simulink model "VMC_14Dof_2024a"  (R2024a)
settings: Solver=FixedStepDiscrete  StartTime=0.0  StopTime=10.0  FixedStep=0.001  RelTol=1e-3
InitFcn:
  | unlinear_14DOF_Parameters
undefined symbols (not defined in the file): Bf, Br, Cp_fl, Cp_fr, Cp_rl, Cp_rr, Cs_f, eta_FMotor, eta_RMotor, f, g, He, Hp, i_fa, i_ra, i_sw, I_tire, Ix, Iy, Iz, ks_f, kw, Lf, Lr, m, mb, mu, mw, r, Sampletime, Standstill_buffer, vx0, vxlim, w0
libraries: simulink x32, slpidlib x6
(part 2 of 5)

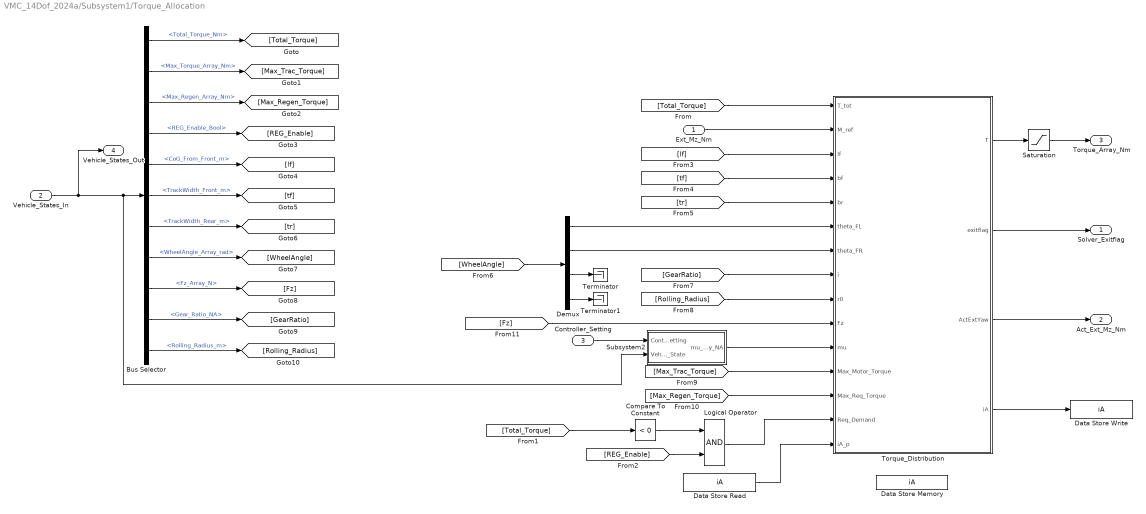
== system VMC_14Dof_2024a/Subsystem1/Torque_Allocation ==
  Ext_Mz_Nm : Inport
  Vehicle_States_In : Inport  Port=2
  Controller_Setting : Inport  Port=3
  Bus Selector : BusSelector  OutputSignals=Torque_Demand.Total_Torque_Nm,Torque_Demand.Max_Torque_Array_Nm,Torque_Demand.Max_Regen_Array_Nm,Torque_Demand.REG_Enable_Bool,Vehicle_Static_Parameter.CoG_From_Front_m,Vehicle_Static_Parameter.TrackWidth_Front_m,Vehicle_Static_Parameter.TrackWidth_Rear_m,WheelAngle.WheelAngle_Array_rad,Tire_Force.Fz_Array_N,Vehicle_Static_Parameter.Gear_Ratio_NA,Vehicle_Static_Parameter.Rolling_Radius_m
  Compare To Constant : simulink/Logic and Bit Operations/Compare To Constant  relop=<  const=0  OutDataTypeStr=boolean
  Data Store Memory : DataStoreMemory  DataStoreName=iA  WriteAfterWriteMsg=warning  InitialValue=[0,0,0,0,0,0,0,0]  ShowAdditionalParam=off  OutDataTypeStr=boolean
  Data Store Read : DataStoreRead  DataStoreName=iA  IndexOptions=Index vector (dialog)  Indices=1  OutputSizes=1
  Data Store Write : DataStoreWrite  DataStoreName=iA  IndexOptions=Index vector (dialog)  Indices=1  OutputSizes=1
  Demux : Demux
  Logical Operator : Logic  AllPortsSameDT=off  OutDataTypeStr=boolean
  Saturation : Saturate  UpperLimit=21  LowerLimit=-21
  Subsystem2 : Subsystem
  Terminator : Terminator
  Terminator1 : Terminator
  Torque_Distribution : MATLAB Function  TreatAsAtomicUnit=on
  Solver_Exitflag : Outport
  Act_Ext_Mz_Nm : Outport  Port=2
  Torque_Array_Nm : Outport  Port=3
  Vehicle_States_Out : Outport  Port=4
  wires:
  [Rolling_Radius] -> Torque_Distribution/9(r0)
  [tr] -> Torque_Distribution/5(br)
  [GearRatio] -> Torque_Distribution/8(i)
  [tf] -> Torque_Distribution/4(bf)
  [lf] -> Torque_Distribution/3(lf)
  [Max_Regen_Torque] -> Torque_Distribution/13(Max_Req_Torque)
  Torque_Distribution/2(exitflag) -> Solver_Exitflag/1
  Demux/1 -> Torque_Distribution/6(theta_FL)
  Demux/2 -> Torque_Distribution/7(theta_FR)
  [Fz] -> Torque_Distribution/10(Fz)
  [Max_Trac_Torque] -> Torque_Distribution/12(Max_Motor_Torque)
  Torque_Distribution/4(iA) -> Data Store Write/1
  Torque_Distribution/1(T) -> Saturation/1
  Data Store Read/1 -> Torque_Distribution/15(iA_p)
  Ext_Mz_Nm/1 -> Torque_Distribution/2(M_ref)
  Subsystem2/1(mu_x_Array_NA) -> Torque_Distribution/11(mu)
  Torque_Distribution/3(ActExtYaw) -> Act_Ext_Mz_Nm/1
  Logical Operator/1 -> Torque_Distribution/14(Req_Demand)
  Compare To Constant/1 -> Logical Operator/1
  [REG_Enable] -> Logical Operator/2
  Vehicle_States_In/1 -> Vehicle_States_Out/1, Subsystem2/2(Vehicle_State), Bus Selector/1
  Bus Selector/1 -> [Total_Torque]  "<Total_Torque_Nm>"
  Bus Selector/2 -> [Max_Trac_Torque]  "<Max_Torque_Array_Nm>"
  Bus Selector/3 -> [Max_Regen_Torque]  "<Max_Regen_Array_Nm>"
  Bus Selector/4 -> [REG_Enable]  "<REG_Enable_Bool>"
  Bus Selector/5 -> [lf]  "<CoG_From_Front_m>"
  Bus Selector/6 -> [tf]  "<TrackWidth_Front_m>"
  Bus Selector/7 -> [tr]  "<TrackWidth_Rear_m>"
  Bus Selector/8 -> [WheelAngle]  "<WheelAngle_Array_rad>"
  Bus Selector/9 -> [Fz]  "<Fz_Array_N>"
  Bus Selector/10 -> [GearRatio]  "<Gear_Ratio_NA>"
  Bus Selector/11 -> [Rolling_Radius]  "<Rolling_Radius_m>"
  [Total_Torque] -> Torque_Distribution/1(T_tot)
  [Total_Torque] -> Compare To Constant/1
  [WheelAngle] -> Demux/1
  Demux/3 -> Terminator/1
  Demux/4 -> Terminator1/1
  Controller_Setting/1 -> Subsystem2/1(Controller_Setting)
  Saturation/1 -> Torque_Array_Nm/1

== system VMC_14Dof_2024a/Subsystem1/Traction_Control ==
  Torque_Array_Nm : Inport
  Vehicle_States_In : Inport  Port=2
  Controller_Setting : Inport  Port=3
  Bus Selector : BusSelector  OutputSignals=TC_Controller.TC_Enable_bool
  LSD_Enable : Subsystem
  LimitedSlipDifferential : Subsystem  Priority=2  TreatAsAtomicUnit=on  RTWFcnName=LimitedSlipDifferential
      settings: RTWSystemCode=Nonreusable function  RTWFcnNameOpts=User specified
  Switch : Switch  Criteria=u2 > Threshold  SaturateOnIntegerOverflow=off  InputSameDT=off
  Cmd_Torque_Nm : Outport
  Vehicle_States_Out : Outport  Port=2
  wires:
  Vehicle_States_In/1 -> Vehicle_States_Out/1, LimitedSlipDifferential/2(Vehicle_States), LSD_Enable/1(Vehicle_States)
  Controller_Setting/1 -> Bus Selector/1, LimitedSlipDifferential/4(Controller_Setting)
  LSD_Enable/1(LSD_Enable) -> LimitedSlipDifferential/3(LSD_Enable)  "LSD_Actv"
  Torque_Array_Nm/1 -> Switch/3, LimitedSlipDifferential/1(Cmd_Torque_Nm)
  Switch/1 -> Cmd_Torque_Nm/1
  LimitedSlipDifferential/1(LSD_Trq) -> Switch/1  "LSD_Trq"
  Bus Selector/1 -> Switch/2  "<TC_Enable_bool>"

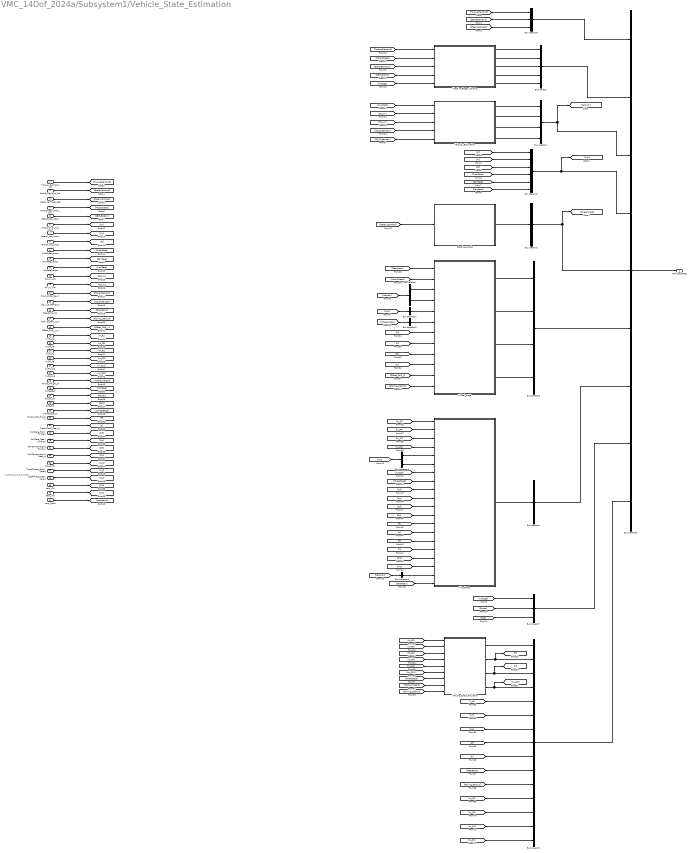
== system VMC_14Dof_2024a/Subsystem1/Vehicle_State_Estimation ==
  note: TireStiffness包含左右轮胎
  Torque_Demand_Pct : Inport  OutDataTypeStr=single
  Brake_Demand_Pct : Inport  Port=2  OutDataTypeStr=single
  SteeringWheel_deg : Inport  Port=3  OutDataTypeStr=single
  MotorSpeed_Array_rpm : Inport  Port=4  OutDataTypeStr=single
  REG_Button_Bool : Inport  Port=5  OutDataTypeStr=boolean
  Longitudinal_Acc_mpss : Inport  Port=6  OutDataTypeStr=single
  Lateral_Acc_mpss : Inport  Port=7  OutDataTypeStr=single
  Vertical_Acc_mpss : Inport  Port=8  OutDataTypeStr=single
  PitchRate_radps : Inport  Port=9  OutDataTypeStr=single
  RollRate_radps : Inport  Port=10  OutDataTypeStr=single
  YawRate_radps : Inport  Port=11  OutDataTypeStr=single
  OS_Vx_kph : Inport  Port=12  OutDataTypeStr=single
  OS_Vy_kph : Inport  Port=13  OutDataTypeStr=single
  OS_X_Distance_m : Inport  Port=14  OutDataTypeStr=single
  OS_Y_Distance_m : Inport  Port=15  OutDataTypeStr=single
  GearRatio_NA : Inport  Port=16  OutDataTypeStr=single
  Rolling_Radius_m : Inport  Port=17  OutDataTypeStr=single
  Offset_CoG_y_m : Inport  Port=18  OutDataTypeStr=single
  m_FL_kg : Inport  Port=19  OutDataTypeStr=single
  m_FR_kg : Inport  Port=20  OutDataTypeStr=single
  m_RL_kg : Inport  Port=21  OutDataTypeStr=single
  m_RR_kg : Inport  Port=22  OutDataTypeStr=single
  m_RL1_kg : Inport  Port=23  OutDataTypeStr=single
  m_RL2_kg : Inport  Port=24  OutDataTypeStr=single
  Table_Height_m : Inport  Port=25  OutDataTypeStr=single
  Voltage_V : Inport  Port=26  OutDataTypeStr=single
  Power_kW : Inport  Port=27  OutDataTypeStr=single
  SoC_Pct : Inport  Port=28  OutDataTypeStr=single
  Wheelbase_m : Inport  Port=29  OutDataTypeStr=single
  TrackWidth_Front_m : Inport  Port=30  OutDataTypeStr=single
  TrackWidth_Rear_m : Inport  Port=31  OutDataTypeStr=single
  RollRate_Front_Nmprad : Inport  Port=32  OutDataTypeStr=single
  RollRate_Rear_Nmprad : Inport  Port=33  OutDataTypeStr=single
  RollCenterHeight_Front_m : Inport  Port=34
  RollCenterHeight_Rear_m : Inport  Port=35
  Izz_kgmm : Inport  Port=36
  TireStiffness_Front_Nprad : Inport  Port=37
  TireStiffness_Rear_Nprad : Inport  Port=38
  Aero_ClA : Inport  Port=39
  Aero_rho : Inport  Port=40
  Aero_Ratio : Inport  Port=41
  Bus Creator : BusCreator  Inputs=5
  Bus Creator1 : BusCreator  Inputs=4
  Bus Creator2 : BusCreator  Inputs=1
  Bus Creator3 : BusCreator  Inputs=4
  Bus Creator4 : BusCreator  Inputs=1
  Bus Creator5 : BusCreator  Inputs=3
  Bus Creator6 : BusCreator  Inputs=6
  Bus Creator7 : BusCreator  Inputs=3
  Bus Creator8 : BusCreator  Inputs=9
  Bus Creator9 : BusCreator  Inputs=15
  Bus Selector : BusSelector  OutputSignals=CoG_Vx_mps,CoG_Vy_mps
  Bus Selector1 : BusSelector  OutputSignals=YawRate_radps
  Bus Selector2 : BusSelector  OutputSignals=WheelAngle_Array_rad
  Bus Selector3 : BusSelector  OutputSignals=CoG_V_mps
  Bus Selector4 : BusSelector  OutputSignals=Longitudinal_Acc_mpss,Lateral_Acc_mpss
  Steering_Angle : Subsystem
  Tire_Force : Subsystem
  Tractive_Regen_Torque : Subsystem
  Vehicle_CoG_Calculation : MATLAB Function  TreatAsAtomicUnit=on
  Velocity_Estimation : Subsystem
  Wheel_State : Subsystem
  Vehicle_States : Outport
  wires:
  Tractive_Regen_Torque/1(Total_Torque_Nm) -> Bus Creator/1  "Total_Torque_Nm"
  Tractive_Regen_Torque/2(Max_Torque_Array_Nm) -> Bus Creator/2  "Max_Torque_Array_Nm"
  Tractive_Regen_Torque/3(Max_Regen_Array_Nm) -> Bus Creator/3  "Max_Regen_Array_Nm"
  Velocity_Estimation/1(CoG_Vx_mps) -> Bus Creator1/1  "CoG_Vx_mps"
  Velocity_Estimation/2(CoG_Vy_mps) -> Bus Creator1/2  "CoG_Vy_mps"
  Velocity_Estimation/3(CoG_V_mps) -> Bus Creator1/3  "CoG_V_mps"
  Velocity_Estimation/4(OS_V_mps) -> Bus Creator1/4  "OS_V_mps"
  Steering_Angle/1(WheelAngle_Array_rad) -> Bus Creator2/1  "WheelAngle_Array_rad"
  Wheel_State/1(Act_WheelSpeed_Array_radps) -> Bus Creator3/1  "Act_WheelSpeed_Array_radps"
  Wheel_State/2(Ref_WheelSpeed_Array_radps) -> Bus Creator3/2  "Ref_WheelSpeed_Array_radps"
  Wheel_State/3(SlipRatio_Array_NA) -> Bus Creator3/3  "SlipRatio_Array_NA"
  Wheel_State/4(Tire_SlipAngle_Array_rad) -> Bus Creator3/4  "Tire_SlipAngle_Array_rad"
  Tire_Force/1(Fz_Array_N) -> Bus Creator4/1  "Fz_Array_N"
  [BrakeDemand] -> Bus Creator5/2  "Brake_Demand_Pct"
  [TorqueDemand] -> Bus Creator5/1  "Torque_Demand_Pct"
  Bus Creator5/1 -> Bus Creator8/1  "Driver_Demand"
  [SteeringWheel] -> Bus Creator5/3  "Steering_Demand_deg"
  Bus Creator/1 -> Bus Creator8/2  "Torque_Demand"
  [Ax] -> Bus Creator6/1  "Longitudinal_Acc_mpss"
  [Ay] -> Bus Creator6/2  "Lateral_Acc_mpss"
  [Az] -> Bus Creator6/3  "Vertical_Acc_mpss"
  [PitchRate] -> Bus Creator6/4  "PitchRate_radps"
  [RollRate] -> Bus Creator6/5  "RollRate_radps"
  [YawRate] -> Bus Creator6/6  "YawRate_radps"
  Bus Creator3/1 -> Bus Creator8/6  "Wheel"
  Bus Creator4/1 -> Bus Creator8/7  "Tire_Force"
  [Voltage] -> Bus Creator7/1  "Voltage_V"
  [Power] -> Bus Creator7/2  "Power_kW"
  [SoC] -> Bus Creator7/3  "SoC_Pct"
  Bus Creator7/1 -> Bus Creator8/8  "Accumulator"
  Bus Creator8/1 -> Vehicle_States/1
  [TorqueDemand] -> Tractive_Regen_Torque/1(Torque_Demand_Pct)
  [BrakeDemand] -> Tractive_Regen_Torque/3(Brake_Demand_Pct)
  [YawRate] -> Velocity_Estimation/1(IMU_YawRate_radps)
  [Voltage] -> Tractive_Regen_Torque/5(HV_Voltage_V)
  Bus Creator1/1 -> [Velocity], Bus Creator8/3  "Vehicle_Velocity"
  Bus Creator6/1 -> [IMU], Bus Creator8/4  "IMU"
  Bus Creator2/1 -> [WheelAngle], Bus Creator8/5  "WheelAngle"
  [Velocity] -> Bus Selector/1
  Bus Selector/1 -> Wheel_State/3(CoG_vx_mps)  "<CoG_Vx_mps>"
  Bus Selector/2 -> Wheel_State/4(CoG_vy_mps)  "<CoG_Vy_mps>"
  [IMU] -> Bus Selector1/1
  Bus Selector1/1 -> Wheel_State/5(Yawrate_radps)  "<YawRate_radps>"
  [WheelAngle] -> Bus Selector2/1
  Bus Selector2/1 -> Wheel_State/6(WheelAngle_Array_rad)  "<WheelAngle_Array_rad>"
  [Velocity] -> Bus Selector3/1
  Bus Selector3/1 -> Tire_Force/19(V_CoG_mps)  "<CoG_V_mps>"
  [IMU] -> Bus Selector4/1
  Bus Selector4/1 -> Tire_Force/5(ax_mpss)  "<Longitudinal_Acc_mpss>"
  Bus Selector4/2 -> Tire_Force/6(ay_mpss)  "<Lateral_Acc_mpss>"
  [SteeringWheel] -> Steering_Angle/1(SteeringWheelAngle_deg)
  [MotorSpeed] -> Tractive_Regen_Torque/2(MotorSpeed_Array_rpm)
  [REG_Button] -> Tractive_Regen_Torque/4(REG_Button_Bool)
  [OS_Vx] -> Velocity_Estimation/2(OS_Vx_kph)
  [OS_Vy] -> Velocity_Estimation/3(OS_Vy_kph)
  [OS_DistanceX] -> Velocity_Estimation/4(OS_X_Distance_m)
  [OS_DistanceY] -> Velocity_Estimation/5(OS_Y_Distance_m)
  [MotorSpeed] -> Wheel_State/2(MotorSpeed_Array_rpm)
  [GearRatio] -> Wheel_State/1(GearRatio_NA)
  [lf] -> Wheel_State/7(lf_m)
  [lr] -> Wheel_State/8(lr_m)
  [tf] -> Wheel_State/9(Trackwidth_Front_m)
  [tr] -> Wheel_State/10(Trackwidth_Rear_m)
  [Offset_CoG_y] -> Wheel_State/11(Offset_CoG_y_m)
  [Rolling_Radius] -> Wheel_State/12(Rolling_Radius_m)
  [m_FL] -> Tire_Force/1(m_FL_kg)
  [m_FR] -> Tire_Force/2(m_FR_kg)
  [m_RL] -> Tire_Force/3(m_RL_kg)
  [m_RR] -> Tire_Force/4(m_RR_kg)
  [h_CoG] -> Tire_Force/7(h_CoG_m)
  [WheelBase] -> Tire_Force/8(Wheelbase_m)
  [tf] -> Tire_Force/13(tf_m)
  [tr] -> Tire_Force/14(tr_m)
  [lf] -> Tire_Force/15(lf_m)
  [lr] -> Tire_Force/16(lr_m)
  [Zrr] -> Tire_Force/12(Zrr_m)
  [Zrf] -> Tire_Force/11(Zrf_m)
  [Krr] -> Tire_Force/10(Krr_Nmprad)
  [Krf] -> Tire_Force/9(Krf_Nmprad)
  [ClA] -> Tire_Force/17(ClA)
  [rho] -> Tire_Force/18(rho)
  [AeroRatio] -> Tire_Force/20(Aero_Ratio)
  Vehicle_CoG_Calculation/4(CoG_Height) -> [h_CoG], Bus Creator9/4  "CoG_Height"
  Vehicle_CoG_Calculation/2(CoG_From_Front) -> [lf], Bus Creator9/2  "CoG_From_Front_m"
  [m_RL1] -> Vehicle_CoG_Calculation/5(m_RL1)
  Vehicle_CoG_Calculation/3(CoG_From_Rear) -> [lr], Bus Creator9/3  "CoG_From_Rear_m"
  [m_FL] -> Vehicle_CoG_Calculation/1(m_FL)
  [Table_Height] -> Vehicle_CoG_Calculation/8(h)
  [Rolling_Radius] -> Vehicle_CoG_Calculation/9(r)
  [m_FR] -> Vehicle_CoG_Calculation/2(m_FR)
  Vehicle_CoG_Calculation/1(Overall_Mass) -> Bus Creator9/1  "Mass_kg"
  [m_RL] -> Vehicle_CoG_Calculation/3(m_RL)
  [WheelBase] -> Vehicle_CoG_Calculation/7(l)
  [m_RR] -> Vehicle_CoG_Calculation/4(m_RR)
  [m_RR1] -> Vehicle_CoG_Calculation/6(m_RR1)
  Bus Creator9/1 -> Bus Creator8/9  "Vehicle_Static_Parameter"
  Torque_Demand_Pct/1 -> [TorqueDemand]
  Brake_Demand_Pct/1 -> [BrakeDemand]
  SteeringWheel_deg/1 -> [SteeringWheel]
  MotorSpeed_Array_rpm/1 -> [MotorSpeed]
  REG_Button_Bool/1 -> [REG_Button]
  Longitudinal_Acc_mpss/1 -> [Ax]
  Lateral_Acc_mpss/1 -> [Ay]
  Vertical_Acc_mpss/1 -> [Az]
  PitchRate_radps/1 -> [PitchRate]
  RollRate_radps/1 -> [RollRate]
  YawRate_radps/1 -> [YawRate]
  OS_Vx_kph/1 -> [OS_Vx]
  OS_Vy_kph/1 -> [OS_Vy]
  OS_X_Distance_m/1 -> [OS_DistanceX]
  OS_Y_Distance_m/1 -> [OS_DistanceY]
  GearRatio_NA/1 -> [GearRatio]
  Rolling_Radius_m/1 -> [Rolling_Radius]
  Offset_CoG_y_m/1 -> [Offset_CoG_y]
  m_FL_kg/1 -> [m_FL]
  m_FR_kg/1 -> [m_FR]
  m_RL_kg/1 -> [m_RL]
  m_RR_kg/1 -> [m_RR]
  m_RL1_kg/1 -> [m_RL1]
  m_RL2_kg/1 -> [m_RR1]
  Table_Height_m/1 -> [Table_Height]
  Voltage_V/1 -> [Voltage]
  Power_kW/1 -> [Power]
  SoC_Pct/1 -> [SoC]
  Wheelbase_m/1 -> [WheelBase]
  TrackWidth_Front_m/1 -> [tf]
  TrackWidth_Rear_m/1 -> [tr]
  RollRate_Front_Nmprad/1 -> [Krf]
  RollRate_Rear_Nmprad/1 -> [Krr]
  RollCenterHeight_Front_m/1 -> [Zrf]
  RollCenterHeight_Rear_m/1 -> [Zrr]
  Aero_ClA/1 -> [ClA]
  Aero_rho/1 -> [rho]
  Aero_Ratio/1 -> [AeroRatio]
  [I_zz] -> Bus Creator9/5  "I_zz_kgmm"
  [K_f] -> Bus Creator9/6  "Kf_Nprad"
  [K_r] -> Bus Creator9/7  "Kr_Nprad"
  TireStiffness_Rear_Nprad/1 -> [K_r]
  TireStiffness_Front_Nprad/1 -> [K_f]
  Izz_kgmm/1 -> [I_zz]
  Tractive_Regen_Torque/4(REG_Enable_Bool) -> Bus Creator/4  "REG_Enable_Bool"
  [tf] -> Bus Creator9/8  "TrackWidth_Front_m"
  [tr] -> Bus Creator9/9  "TrackWidth_Rear_m"
  [GearRatio] -> Bus Creator9/10  "Gear_Ratio_NA"
  [Rolling_Radius] -> Bus Creator9/11  "Rolling_Radius_m"
  [m_FL] -> Bus Creator9/12  "m_FL_kg"
  [m_FR] -> Bus Creator9/13  "m_FR_kg"
  [m_RL] -> Bus Creator9/14  "m_RL_kg"
  [m_RR] -> Bus Creator9/15  "m_RR_kg"
  Tractive_Regen_Torque/5(MotorSpeed_Array_out_rpm) -> Bus Creator/5  "MotorSpeed_Array_rpm"

== system VMC_14Dof_2024a/Subsystem1/YawRate_Controller ==
  Vehicle_States_In : Inport
  Controller_Setting : Inport  Port=2
  CalMz_FB : Subsystem
  CalcMzDes_FF : Subsystem
  Subsystem : Subsystem
  Control_active_flag_bool : Outport
  Ext_Mz_Nm : Outport  Port=2
  Vehicle_States_Out : Outport  Port=3
  wires:
  Vehicle_States_In/1 -> Vehicle_States_Out/1, CalMz_FB/2(Vehicle_States), CalcMzDes_FF/1(Vehicle_States)
  CalcMzDes_FF/3(RefYawRate_radps) -> CalMz_FB/1(RefYawRate_radps)  "Ref_YawRate"
  CalcMzDes_FF/1(Control_active_flag_bool) -> Control_active_flag_bool/1
  CalMz_FB/2(YawRateErr_radps) -> Subsystem/3(YawRateErr_radps)  "YawRate_Error"
  CalcMzDes_FF/2(ExtYawMoment_FF) -> Subsystem/1(ExtYawMoment_FF)  "Ext_Mz_FF"
  CalMz_FB/1(ExtYawMoment_FB) -> Subsystem/2(ExtYawMoment_FB)  "Ext_Mz_FB"
  Subsystem/1(Ext_Mz_Nm) -> Ext_Mz_Nm/1
  Controller_Setting/1 -> Subsystem/4(Controller_Setting), CalMz_FB/3(Controller_Setting)

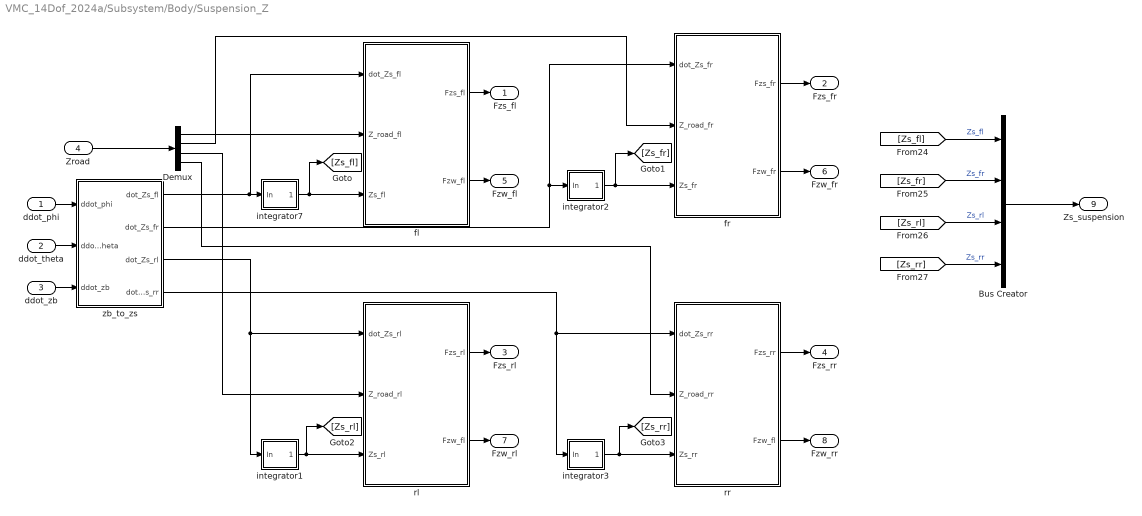
== system VMC_14Dof_2024a/Subsystem/Body/Suspension_Z ==
  ddot_phi : Inport
  ddot_theta : Inport  Port=2
  ddot_zb : Inport  Port=3
  Zroad : Inport  Port=4
  Bus Creator : BusCreator  Inputs=4
  Demux : Demux
  fl : Subsystem
  fr : Subsystem
  integrator1 : Subsystem
  integrator2 : Subsystem
  integrator3 : Subsystem
  integrator7 : Subsystem
  rl : Subsystem
  rr : Subsystem
  zb_to_zs : Subsystem
  Fzs_fl : Outport  VectorParamsAs1DForOutWhenUnconnected=off
  Fzs_fr : Outport  Port=2  VectorParamsAs1DForOutWhenUnconnected=off
  Fzs_rl : Outport  Port=3  VectorParamsAs1DForOutWhenUnconnected=off
  Fzs_rr : Outport  Port=4  VectorParamsAs1DForOutWhenUnconnected=off
  Fzw_fl : Outport  Port=5  VectorParamsAs1DForOutWhenUnconnected=off
  Fzw_fr : Outport  Port=6  VectorParamsAs1DForOutWhenUnconnected=off
  Fzw_rl : Outport  Port=7  VectorParamsAs1DForOutWhenUnconnected=off
  Fzw_rr : Outport  Port=8  VectorParamsAs1DForOutWhenUnconnected=off
  Zs_suspension : Outport  Port=9  VectorParamsAs1DForOutWhenUnconnected=off
  wires:
  ddot_phi/1 -> zb_to_zs/1(ddot_phi)
  ddot_theta/1 -> zb_to_zs/2(ddot_theta)
  ddot_zb/1 -> zb_to_zs/3(ddot_zb)
  fl/1(Fzs_fl) -> Fzs_fl/1
  zb_to_zs/1(dot_Zs_fl) -> fl/1(dot_Zs_fl), integrator7/1(In)
  Zroad/1 -> Demux/1
  integrator7/1(Out) -> [Zs_fl], fl/3(Zs_fl)
  fr/1(Fzs_fr) -> Fzs_fr/1
  zb_to_zs/2(dot_Zs_fr) -> integrator2/1(In), fr/1(dot_Zs_fr)
  Demux/2 -> fr/2(Z_road_fr)
  integrator2/1(Out) -> [Zs_fr], fr/3(Zs_fr)
  fl/2(Fzw_fl) -> Fzw_fl/1
  fr/2(Fzw_fr) -> Fzw_fr/1
  zb_to_zs/3(dot_Zs_rl) -> integrator1/1(In), rl/1(dot_Zs_rl)
  integrator1/1(Out) -> rl/3(Zs_rl), [Zs_rl]
  Demux/3 -> rl/2(Z_road_rl)
  rl/1(Fzs_rl) -> Fzs_rl/1
  rl/2(Fzw_fl) -> Fzw_rl/1
  zb_to_zs/4(dot_Zs_rr) -> integrator3/1(In), rr/1(dot_Zs_rr)
  Demux/4 -> rr/2(Z_road_rr)
  integrator3/1(Out) -> [Zs_rr], rr/3(Zs_rr)
  rr/1(Fzs_rr) -> Fzs_rr/1
  rr/2(Fzw_fl) -> Fzw_rr/1
  Demux/1 -> fl/2(Z_road_fl)
  Bus Creator/1 -> Zs_suspension/1
  [Zs_fr] -> Bus Creator/2  "Zs_fr"
  [Zs_rl] -> Bus Creator/3  "Zs_rl"
  [Zs_rr] -> Bus Creator/4  "Zs_rr"
  [Zs_fl] -> Bus Creator/1  "Zs_fl"

== system VMC_14Dof_2024a/Subsystem/Body/global system transform ==
  vx : Inport
  vy : Inport  Port=2
  wz : Inport  Port=3
  Add : Sum  Inputs=|+-  OutDataTypeStr=single
  Add1 : Sum  Inputs=|++  OutDataTypeStr=single
  Cos : Trigonometry  Operator=cos
  Sin : Trigonometry
  integrator1 : Subsystem
  integrator2 : Subsystem
  integrator8 : Subsystem
  vx*cosr : Product
  vx*sinr : Product
  vy*cosr : Product
  vy*sinr : Product
  x : Outport  VectorParamsAs1DForOutWhenUnconnected=off
  y : Outport  Port=2  VectorParamsAs1DForOutWhenUnconnected=off
  wires:
  Add/1 -> integrator1/1(In)
  Cos/1 -> vy*cosr/2, vx*cosr/2
  vy*sinr/1 -> Add/2
  vx/1 -> vx*sinr/1, vx*cosr/1
  wz/1 -> integrator8/1(wz)
  vy/1 -> vy*sinr/1, vy*cosr/1
  integrator2/1(Out) -> y/1
  integrator1/1(Out) -> x/1
  integrator8/1(Out) -> Cos/1, Sin/1  "r"
  Sin/1 -> vx*sinr/2, vy*sinr/2
  vx*cosr/1 -> Add/1
  vx*sinr/1 -> Add1/1
  Add1/1 -> integrator2/1(In)
  vy*cosr/1 -> Add1/2

== system VMC_14Dof_2024a/Subsystem/Body/integrator1 ==
  In : Inport
  Add : Sum
  Add1 : Sum
  Constant : Constant  Value=Sampletime  OutDataTypeStr=single
  Constant1 : Constant  Value=vx0  OutDataTypeStr=single
  Delay1 : Delay  DelayLength=1  InitialCondition=0
  Divide : Product  Inputs=**
  Saturation : Saturate  UpperLimit=inf  LowerLimit=0
  Out : Outport  VectorParamsAs1DForOutWhenUnconnected=off
  wires:
  In/1 -> Divide/1
  Constant/1 -> Divide/2
  Divide/1 -> Add/1
  Delay1/1 -> Add/2, Add1/2
  Constant1/1 -> Add1/1
  Add1/1 -> Saturation/1
  Add/1 -> Delay1/1
  Saturation/1 -> Out/1

== system VMC_14Dof_2024a/Subsystem/Body/integrator10 ==
  In : Inport
  Add : Sum
  Add1 : Sum
  Constant : Constant  Value=Sampletime  OutDataTypeStr=single
  Constant1 : Constant  Value=0  OutDataTypeStr=single
  Delay1 : Delay  DelayLength=1  InitialCondition=0
  Divide : Product  Inputs=**
  Out : Outport  VectorParamsAs1DForOutWhenUnconnected=off
  wires:
  In/1 -> Divide/1
  Constant/1 -> Divide/2
  Divide/1 -> Add/1
  Delay1/1 -> Add/2, Add1/2
  Constant1/1 -> Add1/1
  Add/1 -> Delay1/1
  Add1/1 -> Out/1

== system VMC_14Dof_2024a/Subsystem/Body/integrator2 ==
  In : Inport
  Add : Sum
  Add1 : Sum
  Constant : Constant  Value=Sampletime  OutDataTypeStr=single
  Constant1 : Constant  Value=0  OutDataTypeStr=single
  Delay1 : Delay  DelayLength=1  InitialCondition=0
  Divide : Product  Inputs=**
  Out : Outport  VectorParamsAs1DForOutWhenUnconnected=off
  wires:
  In/1 -> Divide/1
  Constant/1 -> Divide/2
  Divide/1 -> Add/1
  Delay1/1 -> Add/2, Add1/2
  Constant1/1 -> Add1/1
  Add/1 -> Delay1/1
  Add1/1 -> Out/1

== system VMC_14Dof_2024a/Subsystem/Body/integrator3 ==
  In : Inport
  Add : Sum
  Add1 : Sum
  Constant : Constant  Value=Sampletime  OutDataTypeStr=single
  Constant1 : Constant  Value=0  OutDataTypeStr=single
  Delay1 : Delay  DelayLength=1  InitialCondition=0
  Divide : Product  Inputs=**
  Out : Outport  VectorParamsAs1DForOutWhenUnconnected=off
  wires:
  In/1 -> Divide/1
  Constant/1 -> Divide/2
  Divide/1 -> Add/1
  Delay1/1 -> Add/2, Add1/2
  Constant1/1 -> Add1/1
  Add/1 -> Delay1/1
  Add1/1 -> Out/1

== system VMC_14Dof_2024a/Subsystem/Body/integrator4 ==
  In : Inport
  Add : Sum
  Add1 : Sum
  Constant : Constant  Value=Sampletime  OutDataTypeStr=single
  Constant1 : Constant  Value=0  OutDataTypeStr=single
  Delay1 : Delay  DelayLength=1  InitialCondition=0
  Divide : Product  Inputs=**
  Out : Outport  VectorParamsAs1DForOutWhenUnconnected=off
  wires:
  In/1 -> Divide/1
  Constant/1 -> Divide/2
  Divide/1 -> Add/1
  Delay1/1 -> Add/2, Add1/2
  Constant1/1 -> Add1/1
  Add/1 -> Delay1/1
  Add1/1 -> Out/1

== system VMC_14Dof_2024a/Subsystem/Body/integrator5 ==
  In : Inport
  Add : Sum
  Add1 : Sum
  Constant : Constant  Value=Sampletime  OutDataTypeStr=single
  Constant1 : Constant  Value=0  OutDataTypeStr=single
  Delay1 : Delay  DelayLength=1  InitialCondition=0
  Divide : Product  Inputs=**
  Out : Outport  VectorParamsAs1DForOutWhenUnconnected=off
  wires:
  In/1 -> Divide/1
  Constant/1 -> Divide/2
  Divide/1 -> Add/1
  Delay1/1 -> Add/2, Add1/2
  Constant1/1 -> Add1/1
  Add/1 -> Delay1/1
  Add1/1 -> Out/1

== system VMC_14Dof_2024a/Subsystem/Body/integrator6 ==
  In : Inport
  Add : Sum
  Add1 : Sum
  Constant : Constant  Value=Sampletime  OutDataTypeStr=single
  Constant1 : Constant  Value=0  OutDataTypeStr=single
  Delay1 : Delay  DelayLength=1  InitialCondition=0
  Divide : Product  Inputs=**
  Out : Outport  VectorParamsAs1DForOutWhenUnconnected=off
  wires:
  In/1 -> Divide/1
  Constant/1 -> Divide/2
  Divide/1 -> Add/1
  Delay1/1 -> Add/2, Add1/2
  Constant1/1 -> Add1/1
  Add/1 -> Delay1/1
  Add1/1 -> Out/1

== system VMC_14Dof_2024a/Subsystem/Body/integrator7 ==
  In : Inport
  Add : Sum
  Add1 : Sum
  Constant : Constant  Value=Sampletime  OutDataTypeStr=single
  Constant1 : Constant  Value=0  OutDataTypeStr=single
  Delay1 : Delay  DelayLength=1  InitialCondition=0
  Divide : Product  Inputs=**
  Out : Outport  VectorParamsAs1DForOutWhenUnconnected=off
  wires:
  In/1 -> Divide/1
  Constant/1 -> Divide/2
  Divide/1 -> Add/1
  Delay1/1 -> Add/2, Add1/2
  Constant1/1 -> Add1/1
  Add/1 -> Delay1/1
  Add1/1 -> Out/1

== system VMC_14Dof_2024a/Subsystem/Body/integrator8 ==
  In : Inport
  Add : Sum
  Add1 : Sum
  Constant : Constant  Value=Sampletime  OutDataTypeStr=single
  Constant1 : Constant  Value=0  OutDataTypeStr=single
  Delay1 : Delay  DelayLength=1  InitialCondition=0
  Divide : Product  Inputs=**
  Out : Outport  VectorParamsAs1DForOutWhenUnconnected=off
  wires:
  In/1 -> Divide/1
  Constant/1 -> Divide/2
  Divide/1 -> Add/1
  Delay1/1 -> Add/2, Add1/2
  Constant1/1 -> Add1/1
  Add/1 -> Delay1/1
  Add1/1 -> Out/1

== system VMC_14Dof_2024a/Subsystem/Body/integrator9 ==
  In : Inport
  Add : Sum
  Add1 : Sum
  Constant : Constant  Value=Sampletime  OutDataTypeStr=single
  Constant1 : Constant  Value=0  OutDataTypeStr=single
  Delay1 : Delay  DelayLength=1  InitialCondition=0
  Divide : Product  Inputs=**
  Out : Outport  VectorParamsAs1DForOutWhenUnconnected=off
  wires:
  In/1 -> Divide/1
  Constant/1 -> Divide/2
  Divide/1 -> Add/1
  Delay1/1 -> Add/2, Add1/2
  Constant1/1 -> Add1/1
  Add/1 -> Delay1/1
  Add1/1 -> Out/1

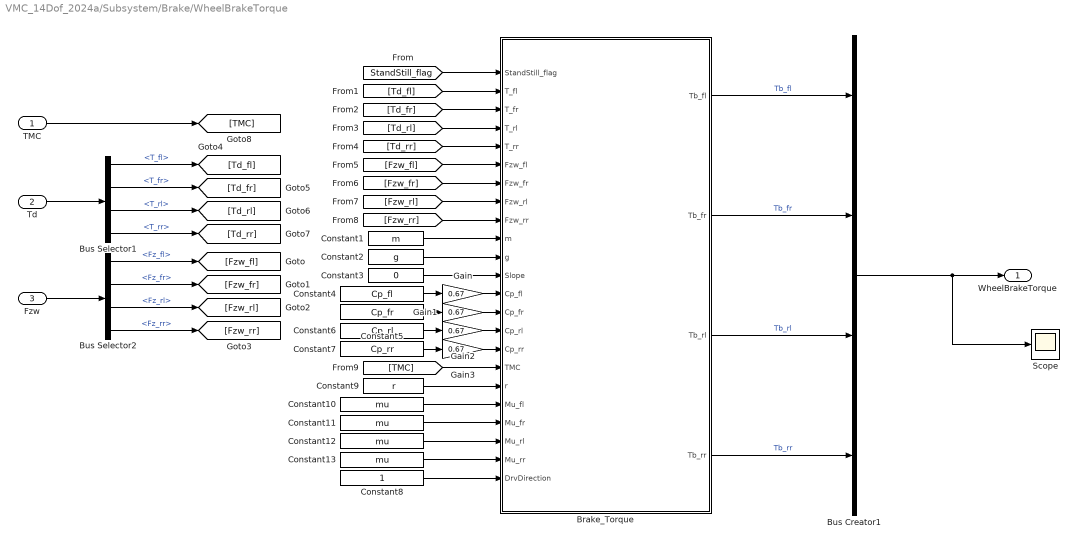
== system VMC_14Dof_2024a/Subsystem/Brake/WheelBrakeTorque ==
  TMC : Inport
  Td : Inport  Port=2
  Fzw : Inport  Port=3
  Brake_Torque : MATLAB Function  TreatAsAtomicUnit=on
  Bus Creator1 : BusCreator  Inputs=4
  Bus Selector1 : BusSelector  OutputSignals=T_fl,T_fr,T_rl,T_rr
  Bus Selector2 : BusSelector  OutputSignals=Fz_fl,Fz_fr,Fz_rl,Fz_rr
  Constant1 : Constant  Value=m  OutDataTypeStr=single
  Constant{10..13} (4 alike) : Constant  Value=mu  OutDataTypeStr=single
  Constant2 : Constant  Value=g  OutDataTypeStr=single
  Constant3 : Constant  Value=0  OutDataTypeStr=single
  Constant4 : Constant  Value=Cp_fl  OutDataTypeStr=single
  Constant5 : Constant  Value=Cp_fr  OutDataTypeStr=single
  Constant6 : Constant  Value=Cp_rl  OutDataTypeStr=single
  Constant7 : Constant  Value=Cp_rr  OutDataTypeStr=single
  Constant8 : Constant  OutDataTypeStr=single
  Constant9 : Constant  Value=r  OutDataTypeStr=single
  Gain{,1..3} (4 alike) : Gain  Gain=0.67  OutDataTypeStr=single
  Scope : Scope
  WheelBrakeTorque : Outport  VectorParamsAs1DForOutWhenUnconnected=off
  wires:
  Bus Creator1/1 -> Scope/1, WheelBrakeTorque/1
  Td/1 -> Bus Selector1/1
  Fzw/1 -> Bus Selector2/1
  Bus Selector2/1 -> [Fzw_fl]  "<Fz_fl>"
  Bus Selector2/3 -> [Fzw_rl]  "<Fz_rl>"
  Bus Selector2/2 -> [Fzw_fr]  "<Fz_fr>"
  Bus Selector2/4 -> [Fzw_rr]  "<Fz_rr>"
  Bus Selector1/1 -> [Td_fl]  "<T_fl>"
  Bus Selector1/2 -> [Td_fr]  "<T_fr>"
  Bus Selector1/3 -> [Td_rl]  "<T_rl>"
  Bus Selector1/4 -> [Td_rr]  "<T_rr>"
  [StandStill_flag] -> Brake_Torque/1(StandStill_flag)
  [Td_fl] -> Brake_Torque/2(T_fl)
  [Td_fr] -> Brake_Torque/3(T_fr)
  [Td_rl] -> Brake_Torque/4(T_rl)
  [Td_rr] -> Brake_Torque/5(T_rr)
  [Fzw_fl] -> Brake_Torque/6(Fzw_fl)
  [Fzw_fr] -> Brake_Torque/7(Fzw_fr)
  [Fzw_rl] -> Brake_Torque/8(Fzw_rl)
  [Fzw_rr] -> Brake_Torque/9(Fzw_rr)
  Constant1/1 -> Brake_Torque/10(m)
  Constant2/1 -> Brake_Torque/11(g)
  Brake_Torque/4(Tb_rr) -> Bus Creator1/4  "Tb_rr"
  Brake_Torque/3(Tb_rl) -> Bus Creator1/3  "Tb_rl"
  Brake_Torque/2(Tb_fr) -> Bus Creator1/2  "Tb_fr"
  Brake_Torque/1(Tb_fl) -> Bus Creator1/1  "Tb_fl"
  TMC/1 -> [TMC]
  [TMC] -> Brake_Torque/17(TMC)
  Constant9/1 -> Brake_Torque/18(r)
  Constant10/1 -> Brake_Torque/19(Mu_fl)
  Constant11/1 -> Brake_Torque/20(Mu_fr)
  Constant12/1 -> Brake_Torque/21(Mu_rl)
  Constant13/1 -> Brake_Torque/22(Mu_rr)
  Constant8/1 -> Brake_Torque/23(DrvDirection)
  Constant3/1 -> Brake_Torque/12(Slope)
  Constant4/1 -> Gain/1
  Gain/1 -> Brake_Torque/13(Cp_fl)
  Constant5/1 -> Gain1/1
  Constant6/1 -> Gain2/1
  Constant7/1 -> Gain3/1
  Gain1/1 -> Brake_Torque/14(Cp_fr)
  Gain2/1 -> Brake_Torque/15(Cp_rl)
  Gain3/1 -> Brake_Torque/16(Cp_rr)

== system VMC_14Dof_2024a/Subsystem/Vehicle State Management/StandStill_thres ==
  In1 : Inport
  Add : Sum  OutDataTypeStr=single
  Add1 : Sum  Inputs=+-  OutDataTypeStr=single
  Compare To Zero : simulink/Logic and Bit Operations/Compare To Zero  relop=<=  OutDataTypeStr=boolean
  Constant : Constant  Value=Standstill_buffer  OutDataTypeStr=single
  Constant1 : Constant  Value=vxlim  OutDataTypeStr=single
  Constant2 : Constant  Value=r  OutDataTypeStr=single
  Divide : Product  Inputs=*/  OutDataTypeStr=single
  Out1 : Outport  VectorParamsAs1DForOutWhenUnconnected=off
  wires:
  Constant/1 -> Add/1
  Constant2/1 -> Divide/2
  Add/1 -> Add1/2
  Add1/1 -> Compare To Zero/1
  Constant1/1 -> Divide/1
  Divide/1 -> Add/2
  In1/1 -> Add1/1
  Compare To Zero/1 -> Out1/1

== system VMC_14Dof_2024a/Subsystem/Vehicle State Management/StandStill_thres1 ==
  In1 : Inport
  Add : Sum  OutDataTypeStr=single
  Add1 : Sum  Inputs=+-  OutDataTypeStr=single
  Compare To Zero : simulink/Logic and Bit Operations/Compare To Zero  relop=<=  OutDataTypeStr=boolean
  Constant : Constant  Value=Standstill_buffer  OutDataTypeStr=single
  Constant1 : Constant  Value=vxlim  OutDataTypeStr=single
  Constant2 : Constant  Value=r  OutDataTypeStr=single
  Divide : Product  Inputs=*/  OutDataTypeStr=single
  Out1 : Outport  VectorParamsAs1DForOutWhenUnconnected=off
  wires:
  Constant/1 -> Add/1
  Constant2/1 -> Divide/2
  Add/1 -> Add1/2
  Add1/1 -> Compare To Zero/1
  Constant1/1 -> Divide/1
  Divide/1 -> Add/2
  In1/1 -> Add1/1
  Compare To Zero/1 -> Out1/1

== system VMC_14Dof_2024a/Subsystem/Vehicle State Management/StandStill_thres2 ==
  In1 : Inport
  Add : Sum  OutDataTypeStr=single
  Add1 : Sum  Inputs=+-  OutDataTypeStr=single
  Compare To Zero : simulink/Logic and Bit Operations/Compare To Zero  relop=<=  OutDataTypeStr=boolean
  Constant : Constant  Value=Standstill_buffer  OutDataTypeStr=single
  Constant1 : Constant  Value=vxlim  OutDataTypeStr=single
  Constant2 : Constant  Value=r  OutDataTypeStr=single
  Divide : Product  Inputs=*/  OutDataTypeStr=single
  Out1 : Outport  VectorParamsAs1DForOutWhenUnconnected=off
  wires:
  Constant/1 -> Add/1
  Constant2/1 -> Divide/2
  Add/1 -> Add1/2
  Add1/1 -> Compare To Zero/1
  Constant1/1 -> Divide/1
  Divide/1 -> Add/2
  In1/1 -> Add1/1
  Compare To Zero/1 -> Out1/1

== system VMC_14Dof_2024a/Subsystem/Vehicle State Management/StandStill_thres3 ==
  In1 : Inport
  Add : Sum  OutDataTypeStr=single
  Add1 : Sum  Inputs=+-  OutDataTypeStr=single
  Compare To Zero : simulink/Logic and Bit Operations/Compare To Zero  relop=<=  OutDataTypeStr=boolean
  Constant : Constant  Value=Standstill_buffer  OutDataTypeStr=single
  Constant1 : Constant  Value=vxlim  OutDataTypeStr=single
  Constant2 : Constant  Value=r  OutDataTypeStr=single
  Divide : Product  Inputs=*/  OutDataTypeStr=single
  Out1 : Outport  VectorParamsAs1DForOutWhenUnconnected=off
  wires:
  Constant/1 -> Add/1
  Constant2/1 -> Divide/2
  Add/1 -> Add1/2
  Add1/1 -> Compare To Zero/1
  Constant1/1 -> Divide/1
  Divide/1 -> Add/2
  In1/1 -> Add1/1
  Compare To Zero/1 -> Out1/1

== system VMC_14Dof_2024a/Subsystem/Vehicle State Management/StandStill_thres4 ==
  In1 : Inport
  Add : Sum  OutDataTypeStr=single
  Add1 : Sum  Inputs=+-  OutDataTypeStr=single
  Compare To Zero : simulink/Logic and Bit Operations/Compare To Zero  relop=<=  OutDataTypeStr=boolean
  Constant : Constant  Value=Standstill_buffer  OutDataTypeStr=single
  Constant1 : Constant  Value=vxlim  OutDataTypeStr=single
  Out1 : Outport  VectorParamsAs1DForOutWhenUnconnected=off
  wires:
  Constant/1 -> Add/1
  Add/1 -> Add1/2
  Add1/1 -> Compare To Zero/1
  Constant1/1 -> Add/2
  In1/1 -> Add1/1
  Compare To Zero/1 -> Out1/1

== system VMC_14Dof_2024a/Subsystem/Wheel/fl ==
  T_fl : Inport
  Fx_fl : Inport  Port=2
  Fz_fl : Inport  Port=3
  Add : Sum  Inputs=+--  OutDataTypeStr=single
  Constant : Constant  Value=I_tire  OutDataTypeStr=single
  Divide : Product  Inputs=*/
  Gain : Gain  Gain=r
  Gain1 : Gain  Gain=r*f
  integrator : Subsystem
  w_fl : Outport  VectorParamsAs1DForOutWhenUnconnected=off
  wires:
  integrator/1(Out) -> w_fl/1
  Divide/1 -> integrator/1(In)  "dot_w"
  Constant/1 -> Divide/2
  Add/1 -> Divide/1
  Gain1/1 -> Add/3
  T_fl/1 -> Add/1
  Fz_fl/1 -> Gain1/1
  Fx_fl/1 -> Gain/1
  Gain/1 -> Add/2

== system VMC_14Dof_2024a/Subsystem/Wheel/fr ==
  T_fr : Inport
  Fx_fr : Inport  Port=2
  Fz_fr : Inport  Port=3
  Add : Sum  Inputs=+--  OutDataTypeStr=single
  Constant : Constant  Value=I_tire  OutDataTypeStr=single
  Divide : Product  Inputs=*/
  Gain : Gain  Gain=r
  Gain1 : Gain  Gain=r*f
  integrator : Subsystem
  w_fr : Outport  VectorParamsAs1DForOutWhenUnconnected=off
  wires:
  Fx_fr/1 -> Gain/1
  Fz_fr/1 -> Gain1/1
  T_fr/1 -> Add/1
  Gain/1 -> Add/2
  Add/1 -> Divide/1
  Constant/1 -> Divide/2
  Divide/1 -> integrator/1(In)  "dot_w"
  integrator/1(Out) -> w_fr/1
  Gain1/1 -> Add/3

== system VMC_14Dof_2024a/Subsystem/Wheel/rl ==
  T_rl : Inport
  Fx_rl : Inport  Port=2
  Fz_rl : Inport  Port=3
  Add : Sum  Inputs=+--  OutDataTypeStr=single
  Constant : Constant  Value=I_tire  OutDataTypeStr=single
  Divide : Product  Inputs=*/
  Gain : Gain  Gain=r
  Gain1 : Gain  Gain=r*f
  integrator : Subsystem
  w_rl : Outport  VectorParamsAs1DForOutWhenUnconnected=off
  wires:
  Fx_rl/1 -> Gain/1
  Fz_rl/1 -> Gain1/1
  T_rl/1 -> Add/1
  Gain/1 -> Add/2
  Add/1 -> Divide/1
  Constant/1 -> Divide/2
  Divide/1 -> integrator/1(In)  "dot_w"
  integrator/1(Out) -> w_rl/1
  Gain1/1 -> Add/3

== system VMC_14Dof_2024a/Subsystem/Wheel/rr ==
  T_rr : Inport
  Fx_rr : Inport  Port=2
  Fz_rr : Inport  Port=3
  Add : Sum  Inputs=+--  OutDataTypeStr=single
  Constant : Constant  Value=I_tire  OutDataTypeStr=single
  Divide : Product  Inputs=*/
  Gain : Gain  Gain=r
  Gain1 : Gain  Gain=r*f
  integrator : Subsystem
  w_rr : Outport  VectorParamsAs1DForOutWhenUnconnected=off
  wires:
  integrator/1(Out) -> w_rr/1
  Divide/1 -> integrator/1(In)  "dot_w"
  Constant/1 -> Divide/2
  Add/1 -> Divide/1
  Gain/1 -> Add/2
  T_rr/1 -> Add/1
  Fz_rr/1 -> Gain1/1
  Fx_rr/1 -> Gain/1
  Gain1/1 -> Add/3

== system VMC_14Dof_2024a/Subsystem/alpha_lamda/alpha ==
  vx : Inport
  vy : Inport  Port=2
  wz : Inport  Port=3
  delta_fl : Inport  Port=4
  delta_fr : Inport  Port=5
  Gain{,1..3} (4 alike) : Gain  Gain=-1
  fl : Subsystem
  fr : Subsystem
  rl : Subsystem
  rr : Subsystem
  alpha_fl : Outport  VectorParamsAs1DForOutWhenUnconnected=off
  alpha_fr : Outport  Port=2  VectorParamsAs1DForOutWhenUnconnected=off
  alpha_rl : Outport  Port=3  VectorParamsAs1DForOutWhenUnconnected=off
  alpha_rr : Outport  Port=4  VectorParamsAs1DForOutWhenUnconnected=off
  wires:
  Gain3/1 -> alpha_rr/1
  rr/1(alpha_rr) -> Gain3/1
  Gain2/1 -> alpha_fr/1
  fr/1(alpha_fr) -> Gain2/1
  Gain1/1 -> alpha_rl/1
  rl/1(alpha_rl) -> Gain1/1
  Gain/1 -> alpha_fl/1
  fl/1(alpha_fl) -> Gain/1
  wz/1 -> fl/3(wz), rr/3(wz), fr/3(wz), rl/3(wz)
  vx/1 -> rr/1(vx), fr/1(vx), fl/1(vx), rl/1(vx)
  vy/1 -> rr/2(vy), fr/2(vy), fl/2(vy), rl/2(vy)
  delta_fl/1 -> fl/4(delta_fl)
  delta_fr/1 -> fr/4(delta_fr)

== system VMC_14Dof_2024a/Subsystem/alpha_lamda/lamda ==
  vx : Inport
  vy : Inport  Port=2
  wz : Inport  Port=3
  delta_fl : Inport  Port=4
  delta_fr : Inport  Port=5
  w_fl : Inport  Port=6
  w_fr : Inport  Port=7
  w_rl : Inport  Port=8
  w_rr : Inport  Port=9
  fl : Subsystem
  fr : Subsystem
  rl : Subsystem
  rr : Subsystem
  lamda_fl : Outport  VectorParamsAs1DForOutWhenUnconnected=off
  lamda_fr : Outport  Port=2  VectorParamsAs1DForOutWhenUnconnected=off
  lamda_rl : Outport  Port=3  VectorParamsAs1DForOutWhenUnconnected=off
  lamda_rr : Outport  Port=4  VectorParamsAs1DForOutWhenUnconnected=off
  wires:
  fl/1(lamda_fl) -> lamda_fl/1
  rl/1(lamda_rl) -> lamda_rl/1
  w_fl/1 -> fl/1(w_fl)
  wz/1 -> rl/2(wz), rr/2(wz), fr/2(wz), fl/2(wz)
  vx/1 -> rl/3(vx), rr/3(vx), fr/3(vx), fl/3(vx)
  vy/1 -> fr/4(vy), fl/4(vy)
  delta_fl/1 -> fl/5(delta_fl)
  delta_fr/1 -> fr/5(delta_fr)
  w_fr/1 -> fr/1(w_fr)
  w_rr/1 -> rr/1(w_rr)
  w_rl/1 -> rl/1(w_rl)
  rr/1(lamda_rr) -> lamda_rr/1
  fr/1(lamda_fr) -> lamda_fr/1

== system VMC_14Dof_2024a/Subsystem1/Power_Limitation/Power_Estimation ==
  Cmd_Torque_Nm : Inport
  Vehicle_States_In : Inport  Port=2
  2-D Lookup Table : Lookup_n-D  BreakpointsForDimension1=[1.3,2.7,5.4,7.9,10.4,12.5,14.4,16,17.4,18.5,19.6]  BreakpointsForDimension2=[500,1000,2000,3000,4000,6000,10000,12000,16000,19000]  BreakpointsForDimension1DataTypeStr=single  BreakpointsForDimension2DataTypeStr=single  Table=reshape([64.37,58.42,44.94,35.59,29.14,24.17,20.41,17.31,14.82,12.81,11.17,71.33,70.84,60.81,51.9,44.78,38.71,33.76,29.4,25.75,22.67,20.05,73.64,77.57,73.35,67.02,61.01,52.22,50.04,45.1,40.67,36.72,33.21,74.7,80.4,78.82,74.26,69.41,64.39,59.65,54.87,50.41,46.3,42.51,75.43,82.01,81.94,78.54,74.57,70.24,65.99,61.55,57.28,53.25,49.44,76.57,83.92,85.43,83.42,80.62,77.3,73.88,70.1,66.34,62.67,59.09,77,85.16,88.2,87.58,85.93,83.73,81.33,78.56,75.7,72.77,69.82,77.08,85.44,88.88,88.65,87.34,85.48,83.42,80.97,78.4,75.75,73.06,77.56,85.97,89.71,89.94,88.86,87.37,85.66,83.56,81.34,79.02,76.63,78.14,86.5,90.44,90.86,90.16,88.98,87.59,85.81,83.91,81.91,79.83],11,10)  TableDataTypeStr=single  IntermediateResultsDataTypeStr=single  InternalRulePriority=Speed  OutDataTypeStr=single  RndMeth=Simplest  FractionDataTypeStr=single
      settings: InputPortMap=u0,u1
  Abs : Abs  SaturateOnIntegerOverflow=off
  Abs1 : Abs  SaturateOnIntegerOverflow=off
  Bus Selector : BusSelector  OutputSignals=Torque_Demand.MotorSpeed_Array_rpm
  MATLAB Function : MATLAB Function  TreatAsAtomicUnit=on
  Est_Power_kW : Outport
  wires:
  Cmd_Torque_Nm/1 -> MATLAB Function/1(Torque), Abs/1
  Abs/1 -> 2-D Lookup Table/1
  Abs1/1 -> 2-D Lookup Table/2
  Vehicle_States_In/1 -> Bus Selector/1
  Bus Selector/1 -> MATLAB Function/3(Speed), Abs1/1  "<MotorSpeed_Array_rpm>"
  2-D Lookup Table/1 -> MATLAB Function/2(Eta)
  MATLAB Function/1(Est_Power) -> Est_Power_kW/1

== system VMC_14Dof_2024a/Subsystem1/Torque_Allocation/Subsystem2 ==
  Controller_Setting : Inport
  Vehicle_State : Inport  Port=2
  Bus Selector : BusSelector  OutputSignals=Tire_Force.Fz_Array_N,Vehicle_Static_Parameter.m_FL_kg,Vehicle_Static_Parameter.m_FR_kg,Vehicle_Static_Parameter.m_RL_kg,Vehicle_Static_Parameter.m_RR_kg,IMU.Lateral_Acc_mpss
  Bus Selector1 : BusSelector  OutputSignals=TC_Controller.Road_Coefficient_NA
  Demux : Demux
  Divide{,1..3} (4 alike) : Product  Inputs=*/*  OutDataTypeStr=single
  Mux : Mux
  mu_x_FL : MATLAB Function  TreatAsAtomicUnit=on
  mu_x_FR : MATLAB Function  TreatAsAtomicUnit=on
  mu_x_RL : MATLAB Function  TreatAsAtomicUnit=on
  mu_x_RR : MATLAB Function  TreatAsAtomicUnit=on
  mu_x_Array_NA : Outport
  wires:
  [m_FL] -> Divide/3
  Vehicle_State/1 -> Bus Selector/1
  Demux/1 -> Divide/2
  Demux/2 -> Divide1/2
  Demux/3 -> Divide2/2
  Demux/4 -> Divide3/2
  [m_FR] -> Divide1/3
  [m_RL] -> Divide2/3
  [m_RR] -> Divide3/3
  Bus Selector1/1 -> mu_x_RR/1(mu), mu_x_RL/1(mu), mu_x_FR/1(mu), mu_x_FL/1(mu)  "<Road_Coefficient_NA>"
  Divide/1 -> mu_x_FL/2(mu_y)
  Divide1/1 -> mu_x_FR/2(mu_y)
  Divide2/1 -> mu_x_RL/2(mu_y)
  Divide3/1 -> mu_x_RR/2(mu_y)
  mu_x_FL/1(mu_x) -> Mux/1
  mu_x_FR/1(mu_x) -> Mux/2
  mu_x_RL/1(mu_x) -> Mux/3
  mu_x_RR/1(mu_x) -> Mux/4
  Mux/1 -> mu_x_Array_NA/1
  [Ay] -> Divide3/1, Divide2/1, Divide1/1, Divide/1
  Bus Selector/1 -> [Fz]  "<Fz_Array_N>"
  Bus Selector/2 -> [m_FL]  "<m_FL_kg>"
  Bus Selector/3 -> [m_FR]  "<m_FR_kg>"
  Bus Selector/4 -> [m_RL]  "<m_RL_kg>"
  Bus Selector/5 -> [m_RR]  "<m_RR_kg>"
  Bus Selector/6 -> [Ay]  "<Lateral_Acc_mpss>"
  [Fz] -> Demux/1
  Controller_Setting/1 -> Bus Selector1/1

== system VMC_14Dof_2024a/Subsystem1/Traction_Control/LSD_Enable ==
  Vehicle_States : Inport
  Bus Selector : BusSelector  OutputSignals=Driver_Demand.Brake_Demand_Pct,Wheel.Act_WheelSpeed_Array_radps,Wheel.SlipRatio_Array_NA
  Demux : Demux
  Demux1 : Demux
  LSD_EnableFL : Subsystem
  LSD_EnableFR : Subsystem
  LSD_EnableRL : Subsystem
  "LSD_EnableRR " : Subsystem
  Mux1 : Mux
  LSD_Enable : Outport
  wires:
  Demux/3 -> LSD_EnableRL/2(WhlSpdActlRL)
  "LSD_EnableRR "/1(LSD_EnableFL) -> Mux1/4  "LSD_EnableRR"
  Demux1/3 -> LSD_EnableRL/3(WhlSpdRefRL)
  Demux/2 -> LSD_EnableFR/2(WhlSpdActlFR)
  LSD_EnableRL/1(LSD_EnableFL) -> Mux1/3  "LSD_EnableRL"
  Demux/1 -> LSD_EnableFL/2(WhlSpdActlFL)
  Bus Selector/3 -> Demux1/1  "<SlipRatio_Array_NA>"
  LSD_EnableFR/1(LSD_EnableFL) -> Mux1/2  "LSD_EnableFR"
  Demux1/4 -> "LSD_EnableRR "/3(WhlSpdRefRR)
  Bus Selector/1 -> LSD_EnableFR/1(BrkDmd), "LSD_EnableRR "/1(BrkDmd), LSD_EnableRL/1(BrkDmd), LSD_EnableFL/1(BrkDmd)  "<Brake_Demand_Pct>"
  Demux1/2 -> LSD_EnableFR/3(WhlSpdRefFR)
  Demux/4 -> "LSD_EnableRR "/2(WhlSpdActlRR)
  Mux1/1 -> LSD_Enable/1  "LSD_Enable"
  Demux1/1 -> LSD_EnableFL/3(WhlSpdRefFL)
  LSD_EnableFL/1(LSD_EnableFL) -> Mux1/1  "LSD_EnableFL"
  Vehicle_States/1 -> Bus Selector/1
  Bus Selector/2 -> Demux/1  "<Act_WheelSpeed_Array_radps>"

== system VMC_14Dof_2024a/Subsystem1/Traction_Control/LimitedSlipDifferential ==
  Cmd_Torque_Nm : Inport
  Vehicle_States : Inport  Port=2
  LSD_Enable : Inport  Port=3
  Controller_Setting : Inport  Port=4
  Demux : Demux
  LSD_Ctrl : Subsystem
  Mux : Mux
  PID_CtrlFL : Subsystem
  PID_CtrlFR : Subsystem
  PID_CtrlRL : Subsystem
  PID_CtrlRR : Subsystem
  Subsystem : Subsystem
  LSD_Trq : Outport  VectorParamsAs1DForOutWhenUnconnected=off
  wires:
  PID_CtrlFL/1(LSD_TrqFL) -> Mux/1  "LSD_TrqFL"
  PID_CtrlRL/1(LSD_TrqRL) -> Mux/3  "LSD_TrqRL"
  PID_CtrlRR/1(LSD_TrqRR) -> Mux/4  "LSD_TrqRR"
  Cmd_Torque_Nm/1 -> Demux/1
  Demux/1 -> PID_CtrlFL/2(EDS_TrqFL)  "TrqFL"
  Demux/2 -> PID_CtrlFR/2(EDS_TrqFR)  "TrqFR"
  Demux/3 -> PID_CtrlRL/2(EDS_TrqRL)  "TrqRL"
  Demux/4 -> PID_CtrlRR/2(EDS_TrqRR)  "TrqRR"
  LSD_Ctrl/1(LSD_CtrlFL) -> PID_CtrlFL/1(LSD_CtrlFL)
  LSD_Ctrl/2(LSD_CtrlFR) -> PID_CtrlFR/1(LSD_CtrlFR)
  LSD_Ctrl/3(LSD_CtrlRL) -> PID_CtrlRL/1(LSD_CtrlRL)
  LSD_Ctrl/4(LSD_CtrlRR) -> PID_CtrlRR/1(LSD_CtrlRR)
  Mux/1 -> LSD_Trq/1  "LSD_Trq"
  PID_CtrlFR/1(LSD_TrqFR) -> Mux/2  "LSD_TrqFR"
  Vehicle_States/1 -> LSD_Ctrl/1(Vehicle_States)
  LSD_Enable/1 -> Subsystem/1(LSD_Enable), LSD_Ctrl/2(LSD_Enable)
  Controller_Setting/1 -> Subsystem/2(Controller_Setting)
  Subsystem/1(PID_Setting) -> PID_CtrlRR/3(PID_Setting), PID_CtrlRL/3(PID_Setting), PID_CtrlFR/3(PID_Setting), PID_CtrlFL/3(PID_Setting)
